simulink model "positionControl"  (Simulink 8.3)
settings: Solver=FixedStepDiscrete  StartTime=0.0  StopTime=simulationTime  FixedStep=Ts  RelTol=1e-3
InitFcn:
  | initPositionControl;
undefined symbols (not defined in the file or in its folder): amplitudesOscillations, frequenciesOscillations
undefined symbols (not defined in the file): localName, robotName, Ts
libraries: WBCLibrary x6
settings Model: Creator=daniele  LastModifiedBy=daniele
settings DataIOCC: SignalLoggingSaveFormat=Dataset
settings OptimizationCC: ExpressionDepthLimit=2147483647
settings DebuggingCC: FcnCallInpInsideContextMsg=EnableAllAsWarning
settings SFSimCC: SimParseCustomCode=off

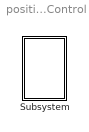
== system positionControl ==
  Subsystem : Subsystem  mask{robotName=robotName, Ts=Ts, localName=localName}
      mask prompts: robotName "robot name"; localName "module name"

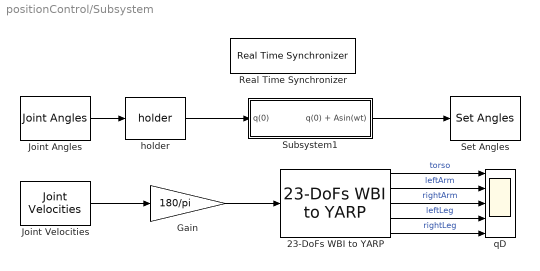
== system positionControl/Subsystem ==
  23-DoFs WBI to YARP : WBCLibrary/Utilities/23-DoFs WBI to YARP
  Gain : Gain  Gain=180/pi
  Joint Angles : WBCLibrary/wholeBodyStates/Joint Angles  robotName=robotName  localName=localName
  Joint Velocities : WBCLibrary/wholeBodyStates/Joint Velocities  robotName=robotName  localName=localName
  Real Time Synchronizer : WBCLibrary/Utilities/Real Time Synchronizer  Priority=-10  threadPeriod=Ts
  Set Angles : WBCLibrary/wholeBodyActuators/Set Angles  val=5  robotName=robotName  localName=localName
  Subsystem1 : Subsystem
  "holder " : WBCLibrary/Utilities/holder 
  qD : Scope  NumInputPorts=5
      settings: ShowLegends=on  TimeRange=5  YMin=-50~-50~-50~-100~-100  YMax=100~50~50~100~100
  wires:
  Joint Angles/1 -> "holder "/1
  "holder "/1 -> Subsystem1/1(q(0))
  Subsystem1/1(q(0) + Asin(wt)) -> Set Angles/1
  Joint Velocities/1 -> Gain/1
  23-DoFs WBI to YARP/4 -> qD/4  "leftLeg"
  23-DoFs WBI to YARP/5 -> qD/5  "rightLeg"
  23-DoFs WBI to YARP/1 -> qD/1  "torso"
  23-DoFs WBI to YARP/2 -> qD/2  "leftArm"
  23-DoFs WBI to YARP/3 -> qD/3  "rightArm"
  Gain/1 -> 23-DoFs WBI to YARP/1

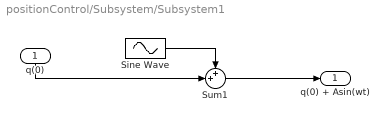
== system positionControl/Subsystem/Subsystem1 ==
  q(0) : Inport
  Sine Wave : Sin  Amplitude=amplitudesOscillations*pi/180  Frequency=frequenciesOscillations*2*pi  SampleTime=0
  Sum1 : Sum  Inputs=++|
  q(0) + Asin(wt) : Outport
  wires:
  q(0)/1 -> Sum1/2
  Sine Wave/1 -> Sum1/1
  Sum1/1 -> q(0) + Asin(wt)/1
